simulink library "MIL_Test"  (Simulink 7.0)
values from neighbouring files (symbols this model uses):
  TID = min('TI' == AFT(1:2))    [PAS_callback.m]    (also in PSTID_callback.m = [block '/TID'])
undefined symbols (not defined in the file or in its folder): getdatatypespecs, slcm, StepSize
libraries: simulink x71, MIL_Test x6
(part 5 of 11)

== system MIL_Test/Test Data/Feature generation/Generate timed limited decrease/Subsystem/Subsystem40 ==
  In1 : Inport  OutDataType=sfix(16)  OutScaling=2^0
  In2 : Inport  Port=2  OutDataType=sfix(16)  OutScaling=2^0
  In3 : Inport  Port=3  OutDataType=sfix(16)  OutScaling=2^0
  Output1 : Sum  Inputs=|+-+  OutDataType=sfix(16)  OutScaling=2^0  SaturateOnIntegerOverflow=on  InputSameDT=on
  RO : RelationalOperator  Operator=<  LogicOutDataTypeMode=boolean
  Switch : Switch  Criteria=u2 > Threshold
  Out1 : Outport  OutDataType=sfix(16)  OutScaling=2^0
  wires:
  In3/1 -> Output1/3
  Output1/1 -> Switch/1
  RO/1 -> Switch/2
  Switch/1 -> Out1/1
  In2/1 -> RO/1, Output1/1, Switch/3  "U(k)"
  In1/1 -> RO/2, Output1/2

== system MIL_Test/Test Data/Feature generation/Generate timed limited decrease/Subsystem/Subsystem41 ==
  In1 : Inport  OutDataType=sfix(16)  OutScaling=2^0
  In2 : Inport  Port=2  OutDataType=sfix(16)  OutScaling=2^0
  In3 : Inport  Port=3  OutDataType=sfix(16)  OutScaling=2^0
  Output1 : Sum  Inputs=|+-+  OutDataType=sfix(16)  OutScaling=2^0  SaturateOnIntegerOverflow=on  InputSameDT=on
  RO : RelationalOperator  Operator=<  LogicOutDataTypeMode=boolean
  Switch : Switch  Criteria=u2 > Threshold
  Out1 : Outport  OutDataType=sfix(16)  OutScaling=2^0
  wires:
  In3/1 -> Output1/3
  Output1/1 -> Switch/1
  RO/1 -> Switch/2
  Switch/1 -> Out1/1
  In2/1 -> RO/1, Output1/1, Switch/3  "U(k)"
  In1/1 -> RO/2, Output1/2

== system MIL_Test/Test Data/Feature generation/Generate timed limited decrease/Subsystem/Subsystem42 ==
  In1 : Inport  OutDataType=sfix(16)  OutScaling=2^0
  In2 : Inport  Port=2  OutDataType=sfix(16)  OutScaling=2^0
  In3 : Inport  Port=3  OutDataType=sfix(16)  OutScaling=2^0
  Output1 : Sum  Inputs=|+-+  OutDataType=sfix(16)  OutScaling=2^0  SaturateOnIntegerOverflow=on  InputSameDT=on
  RO : RelationalOperator  Operator=<  LogicOutDataTypeMode=boolean
  Switch : Switch  Criteria=u2 > Threshold
  Out1 : Outport  OutDataType=sfix(16)  OutScaling=2^0
  wires:
  In3/1 -> Output1/3
  Output1/1 -> Switch/1
  RO/1 -> Switch/2
  Switch/1 -> Out1/1
  In2/1 -> RO/1, Output1/1, Switch/3  "U(k)"
  In1/1 -> RO/2, Output1/2

== system MIL_Test/Test Data/Feature generation/Generate timed limited decrease/Subsystem/Subsystem43 ==
  In1 : Inport  OutDataType=sfix(16)  OutScaling=2^0
  In2 : Inport  Port=2  OutDataType=sfix(16)  OutScaling=2^0
  In3 : Inport  Port=3  OutDataType=sfix(16)  OutScaling=2^0
  Output1 : Sum  Inputs=|+-+  OutDataType=sfix(16)  OutScaling=2^0  SaturateOnIntegerOverflow=on  InputSameDT=on
  RO : RelationalOperator  Operator=<  LogicOutDataTypeMode=boolean
  Switch : Switch  Criteria=u2 > Threshold
  Out1 : Outport  OutDataType=sfix(16)  OutScaling=2^0
  wires:
  In3/1 -> Output1/3
  Output1/1 -> Switch/1
  RO/1 -> Switch/2
  Switch/1 -> Out1/1
  In2/1 -> RO/1, Output1/1, Switch/3  "U(k)"
  In1/1 -> RO/2, Output1/2

== system MIL_Test/Test Data/Feature generation/Generate timed limited decrease/Subsystem/Subsystem44 ==
  In1 : Inport  OutDataType=sfix(16)  OutScaling=2^0
  In2 : Inport  Port=2  OutDataType=sfix(16)  OutScaling=2^0
  In3 : Inport  Port=3  OutDataType=sfix(16)  OutScaling=2^0
  Output1 : Sum  Inputs=|+-+  OutDataType=sfix(16)  OutScaling=2^0  SaturateOnIntegerOverflow=on  InputSameDT=on
  RO : RelationalOperator  Operator=<  LogicOutDataTypeMode=boolean
  Switch : Switch  Criteria=u2 > Threshold
  Out1 : Outport  OutDataType=sfix(16)  OutScaling=2^0
  wires:
  In3/1 -> Output1/3
  Output1/1 -> Switch/1
  RO/1 -> Switch/2
  Switch/1 -> Out1/1
  In2/1 -> RO/1, Output1/1, Switch/3  "U(k)"
  In1/1 -> RO/2, Output1/2

== system MIL_Test/Test Data/Feature generation/Generate timed limited decrease/Subsystem/Subsystem45 ==
  In1 : Inport  OutDataType=sfix(16)  OutScaling=2^0
  In2 : Inport  Port=2  OutDataType=sfix(16)  OutScaling=2^0
  In3 : Inport  Port=3  OutDataType=sfix(16)  OutScaling=2^0
  Output1 : Sum  Inputs=|+-+  OutDataType=sfix(16)  OutScaling=2^0  SaturateOnIntegerOverflow=on  InputSameDT=on
  RO : RelationalOperator  Operator=<  LogicOutDataTypeMode=boolean
  Switch : Switch  Criteria=u2 > Threshold
  Out1 : Outport  OutDataType=sfix(16)  OutScaling=2^0
  wires:
  In3/1 -> Output1/3
  Output1/1 -> Switch/1
  RO/1 -> Switch/2
  Switch/1 -> Out1/1
  In2/1 -> RO/1, Output1/1, Switch/3  "U(k)"
  In1/1 -> RO/2, Output1/2

== system MIL_Test/Test Data/Feature generation/Generate timed limited decrease/Subsystem/Subsystem46 ==
  In1 : Inport  OutDataType=sfix(16)  OutScaling=2^0
  In2 : Inport  Port=2  OutDataType=sfix(16)  OutScaling=2^0
  In3 : Inport  Port=3  OutDataType=sfix(16)  OutScaling=2^0
  Output1 : Sum  Inputs=|+-+  OutDataType=sfix(16)  OutScaling=2^0  SaturateOnIntegerOverflow=on  InputSameDT=on
  RO : RelationalOperator  Operator=<  LogicOutDataTypeMode=boolean
  Switch : Switch  Criteria=u2 > Threshold
  Out1 : Outport  OutDataType=sfix(16)  OutScaling=2^0
  wires:
  In3/1 -> Output1/3
  Output1/1 -> Switch/1
  RO/1 -> Switch/2
  Switch/1 -> Out1/1
  In2/1 -> RO/1, Output1/1, Switch/3  "U(k)"
  In1/1 -> RO/2, Output1/2

== system MIL_Test/Test Data/Feature generation/Generate timed limited decrease/Subsystem/Subsystem47 ==
  In1 : Inport  OutDataType=sfix(16)  OutScaling=2^0
  In2 : Inport  Port=2  OutDataType=sfix(16)  OutScaling=2^0
  In3 : Inport  Port=3  OutDataType=sfix(16)  OutScaling=2^0
  Output1 : Sum  Inputs=|+-+  OutDataType=sfix(16)  OutScaling=2^0  SaturateOnIntegerOverflow=on  InputSameDT=on
  RO : RelationalOperator  Operator=<  LogicOutDataTypeMode=boolean
  Switch : Switch  Criteria=u2 > Threshold
  Out1 : Outport  OutDataType=sfix(16)  OutScaling=2^0
  wires:
  In3/1 -> Output1/3
  Output1/1 -> Switch/1
  RO/1 -> Switch/2
  Switch/1 -> Out1/1
  In2/1 -> RO/1, Output1/1, Switch/3  "U(k)"
  In1/1 -> RO/2, Output1/2

== system MIL_Test/Test Data/Feature generation/Generate timed limited decrease/Subsystem/Subsystem48 ==
  In1 : Inport  OutDataType=sfix(16)  OutScaling=2^0
  In2 : Inport  Port=2  OutDataType=sfix(16)  OutScaling=2^0
  In3 : Inport  Port=3  OutDataType=sfix(16)  OutScaling=2^0
  Output1 : Sum  Inputs=|+-+  OutDataType=sfix(16)  OutScaling=2^0  SaturateOnIntegerOverflow=on  InputSameDT=on
  RO : RelationalOperator  Operator=<  LogicOutDataTypeMode=boolean
  Switch : Switch  Criteria=u2 > Threshold
  Out1 : Outport  OutDataType=sfix(16)  OutScaling=2^0
  wires:
  In3/1 -> Output1/3
  Output1/1 -> Switch/1
  RO/1 -> Switch/2
  Switch/1 -> Out1/1
  In2/1 -> RO/1, Output1/1, Switch/3  "U(k)"
  In1/1 -> RO/2, Output1/2

== system MIL_Test/Test Data/Feature generation/Generate timed limited decrease/Subsystem/Subsystem49 ==
  In1 : Inport  OutDataType=sfix(16)  OutScaling=2^0
  In2 : Inport  Port=2  OutDataType=sfix(16)  OutScaling=2^0
  In3 : Inport  Port=3  OutDataType=sfix(16)  OutScaling=2^0
  Output1 : Sum  Inputs=|+-+  OutDataType=sfix(16)  OutScaling=2^0  SaturateOnIntegerOverflow=on  InputSameDT=on
  RO : RelationalOperator  Operator=<  LogicOutDataTypeMode=boolean
  Switch : Switch  Criteria=u2 > Threshold
  Out1 : Outport  OutDataType=sfix(16)  OutScaling=2^0
  wires:
  In3/1 -> Output1/3
  Output1/1 -> Switch/1
  RO/1 -> Switch/2
  Switch/1 -> Out1/1
  In2/1 -> RO/1, Output1/1, Switch/3  "U(k)"
  In1/1 -> RO/2, Output1/2

== system MIL_Test/Test Data/Feature generation/Generate timed limited decrease/Subsystem/Subsystem5 ==
  In1 : Inport  OutDataType=sfix(16)  OutScaling=2^0
  In2 : Inport  Port=2  OutDataType=sfix(16)  OutScaling=2^0
  In3 : Inport  Port=3  OutDataType=sfix(16)  OutScaling=2^0
  Output1 : Sum  Inputs=|+-+  OutDataType=sfix(16)  OutScaling=2^0  SaturateOnIntegerOverflow=on  InputSameDT=on
  RO : RelationalOperator  Operator=<  LogicOutDataTypeMode=boolean
  Switch : Switch  Criteria=u2 > Threshold
  Out1 : Outport  OutDataType=sfix(16)  OutScaling=2^0
  wires:
  In3/1 -> Output1/3
  Output1/1 -> Switch/1
  RO/1 -> Switch/2
  Switch/1 -> Out1/1
  In2/1 -> RO/1, Output1/1, Switch/3  "U(k)"
  In1/1 -> RO/2, Output1/2

== system MIL_Test/Test Data/Feature generation/Generate timed limited decrease/Subsystem/Subsystem50 ==
  In1 : Inport  OutDataType=sfix(16)  OutScaling=2^0
  In2 : Inport  Port=2  OutDataType=sfix(16)  OutScaling=2^0
  In3 : Inport  Port=3  OutDataType=sfix(16)  OutScaling=2^0
  Output1 : Sum  Inputs=|+-+  OutDataType=sfix(16)  OutScaling=2^0  SaturateOnIntegerOverflow=on  InputSameDT=on
  RO : RelationalOperator  Operator=<  LogicOutDataTypeMode=boolean
  Switch : Switch  Criteria=u2 > Threshold
  Out1 : Outport  OutDataType=sfix(16)  OutScaling=2^0
  wires:
  In3/1 -> Output1/3
  Output1/1 -> Switch/1
  RO/1 -> Switch/2
  Switch/1 -> Out1/1
  In2/1 -> RO/1, Output1/1, Switch/3  "U(k)"
  In1/1 -> RO/2, Output1/2

== system MIL_Test/Test Data/Feature generation/Generate timed limited decrease/Subsystem/Subsystem51 ==
  In1 : Inport  OutDataType=sfix(16)  OutScaling=2^0
  In2 : Inport  Port=2  OutDataType=sfix(16)  OutScaling=2^0
  In3 : Inport  Port=3  OutDataType=sfix(16)  OutScaling=2^0
  Output1 : Sum  Inputs=|+-+  OutDataType=sfix(16)  OutScaling=2^0  SaturateOnIntegerOverflow=on  InputSameDT=on
  RO : RelationalOperator  Operator=<  LogicOutDataTypeMode=boolean
  Switch : Switch  Criteria=u2 > Threshold
  Out1 : Outport  OutDataType=sfix(16)  OutScaling=2^0
  wires:
  In3/1 -> Output1/3
  Output1/1 -> Switch/1
  RO/1 -> Switch/2
  Switch/1 -> Out1/1
  In2/1 -> RO/1, Output1/1, Switch/3  "U(k)"
  In1/1 -> RO/2, Output1/2

== system MIL_Test/Test Data/Feature generation/Generate timed limited decrease/Subsystem/Subsystem52 ==
  In1 : Inport  OutDataType=sfix(16)  OutScaling=2^0
  In2 : Inport  Port=2  OutDataType=sfix(16)  OutScaling=2^0
  In3 : Inport  Port=3  OutDataType=sfix(16)  OutScaling=2^0
  Output1 : Sum  Inputs=|+-+  OutDataType=sfix(16)  OutScaling=2^0  SaturateOnIntegerOverflow=on  InputSameDT=on
  RO : RelationalOperator  Operator=<  LogicOutDataTypeMode=boolean
  Switch : Switch  Criteria=u2 > Threshold
  Out1 : Outport  OutDataType=sfix(16)  OutScaling=2^0
  wires:
  In3/1 -> Output1/3
  Output1/1 -> Switch/1
  RO/1 -> Switch/2
  Switch/1 -> Out1/1
  In2/1 -> RO/1, Output1/1, Switch/3  "U(k)"
  In1/1 -> RO/2, Output1/2

== system MIL_Test/Test Data/Feature generation/Generate timed limited decrease/Subsystem/Subsystem53 ==
  In1 : Inport  OutDataType=sfix(16)  OutScaling=2^0
  In2 : Inport  Port=2  OutDataType=sfix(16)  OutScaling=2^0
  In3 : Inport  Port=3  OutDataType=sfix(16)  OutScaling=2^0
  Output1 : Sum  Inputs=|+-+  OutDataType=sfix(16)  OutScaling=2^0  SaturateOnIntegerOverflow=on  InputSameDT=on
  RO : RelationalOperator  Operator=<  LogicOutDataTypeMode=boolean
  Switch : Switch  Criteria=u2 > Threshold
  Out1 : Outport  OutDataType=sfix(16)  OutScaling=2^0
  wires:
  In3/1 -> Output1/3
  Output1/1 -> Switch/1
  RO/1 -> Switch/2
  Switch/1 -> Out1/1
  In2/1 -> RO/1, Output1/1, Switch/3  "U(k)"
  In1/1 -> RO/2, Output1/2

== system MIL_Test/Test Data/Feature generation/Generate timed limited decrease/Subsystem/Subsystem54 ==
  In1 : Inport  OutDataType=sfix(16)  OutScaling=2^0
  In2 : Inport  Port=2  OutDataType=sfix(16)  OutScaling=2^0
  In3 : Inport  Port=3  OutDataType=sfix(16)  OutScaling=2^0
  Output1 : Sum  Inputs=|+-+  OutDataType=sfix(16)  OutScaling=2^0  SaturateOnIntegerOverflow=on  InputSameDT=on
  RO : RelationalOperator  Operator=<  LogicOutDataTypeMode=boolean
  Switch : Switch  Criteria=u2 > Threshold
  Out1 : Outport  OutDataType=sfix(16)  OutScaling=2^0
  wires:
  In3/1 -> Output1/3
  Output1/1 -> Switch/1
  RO/1 -> Switch/2
  Switch/1 -> Out1/1
  In2/1 -> RO/1, Output1/1, Switch/3  "U(k)"
  In1/1 -> RO/2, Output1/2

== system MIL_Test/Test Data/Feature generation/Generate timed limited decrease/Subsystem/Subsystem55 ==
  In1 : Inport  OutDataType=sfix(16)  OutScaling=2^0
  In2 : Inport  Port=2  OutDataType=sfix(16)  OutScaling=2^0
  In3 : Inport  Port=3  OutDataType=sfix(16)  OutScaling=2^0
  Output1 : Sum  Inputs=|+-+  OutDataType=sfix(16)  OutScaling=2^0  SaturateOnIntegerOverflow=on  InputSameDT=on
  RO : RelationalOperator  Operator=<  LogicOutDataTypeMode=boolean
  Switch : Switch  Criteria=u2 > Threshold
  Out1 : Outport  OutDataType=sfix(16)  OutScaling=2^0
  wires:
  In3/1 -> Output1/3
  Output1/1 -> Switch/1
  RO/1 -> Switch/2
  Switch/1 -> Out1/1
  In2/1 -> RO/1, Output1/1, Switch/3  "U(k)"
  In1/1 -> RO/2, Output1/2

== system MIL_Test/Test Data/Feature generation/Generate timed limited decrease/Subsystem/Subsystem56 ==
  In1 : Inport  OutDataType=sfix(16)  OutScaling=2^0
  In2 : Inport  Port=2  OutDataType=sfix(16)  OutScaling=2^0
  In3 : Inport  Port=3  OutDataType=sfix(16)  OutScaling=2^0
  Output1 : Sum  Inputs=|+-+  OutDataType=sfix(16)  OutScaling=2^0  SaturateOnIntegerOverflow=on  InputSameDT=on
  RO : RelationalOperator  Operator=<  LogicOutDataTypeMode=boolean
  Switch : Switch  Criteria=u2 > Threshold
  Out1 : Outport  OutDataType=sfix(16)  OutScaling=2^0
  wires:
  In3/1 -> Output1/3
  Output1/1 -> Switch/1
  RO/1 -> Switch/2
  Switch/1 -> Out1/1
  In2/1 -> RO/1, Output1/1, Switch/3  "U(k)"
  In1/1 -> RO/2, Output1/2

== system MIL_Test/Test Data/Feature generation/Generate timed limited decrease/Subsystem/Subsystem57 ==
  In1 : Inport  OutDataType=sfix(16)  OutScaling=2^0
  In2 : Inport  Port=2  OutDataType=sfix(16)  OutScaling=2^0
  In3 : Inport  Port=3  OutDataType=sfix(16)  OutScaling=2^0
  Output1 : Sum  Inputs=|+-+  OutDataType=sfix(16)  OutScaling=2^0  SaturateOnIntegerOverflow=on  InputSameDT=on
  RO : RelationalOperator  Operator=<  LogicOutDataTypeMode=boolean
  Switch : Switch  Criteria=u2 > Threshold
  Out1 : Outport  OutDataType=sfix(16)  OutScaling=2^0
  wires:
  In3/1 -> Output1/3
  Output1/1 -> Switch/1
  RO/1 -> Switch/2
  Switch/1 -> Out1/1
  In2/1 -> RO/1, Output1/1, Switch/3  "U(k)"
  In1/1 -> RO/2, Output1/2

== system MIL_Test/Test Data/Feature generation/Generate timed limited decrease/Subsystem/Subsystem58 ==
  In1 : Inport  OutDataType=sfix(16)  OutScaling=2^0
  In2 : Inport  Port=2  OutDataType=sfix(16)  OutScaling=2^0
  In3 : Inport  Port=3  OutDataType=sfix(16)  OutScaling=2^0
  Output1 : Sum  Inputs=|+-+  OutDataType=sfix(16)  OutScaling=2^0  SaturateOnIntegerOverflow=on  InputSameDT=on
  RO : RelationalOperator  Operator=<  LogicOutDataTypeMode=boolean
  Switch : Switch  Criteria=u2 > Threshold
  Out1 : Outport  OutDataType=sfix(16)  OutScaling=2^0
  wires:
  In3/1 -> Output1/3
  Output1/1 -> Switch/1
  RO/1 -> Switch/2
  Switch/1 -> Out1/1
  In2/1 -> RO/1, Output1/1, Switch/3  "U(k)"
  In1/1 -> RO/2, Output1/2

== system MIL_Test/Test Data/Feature generation/Generate timed limited decrease/Subsystem/Subsystem59 ==
  In1 : Inport  OutDataType=sfix(16)  OutScaling=2^0
  In2 : Inport  Port=2  OutDataType=sfix(16)  OutScaling=2^0
  In3 : Inport  Port=3  OutDataType=sfix(16)  OutScaling=2^0
  Output1 : Sum  Inputs=|+-+  OutDataType=sfix(16)  OutScaling=2^0  SaturateOnIntegerOverflow=on  InputSameDT=on
  RO : RelationalOperator  Operator=<  LogicOutDataTypeMode=boolean
  Switch : Switch  Criteria=u2 > Threshold
  Out1 : Outport  OutDataType=sfix(16)  OutScaling=2^0
  wires:
  In3/1 -> Output1/3
  Output1/1 -> Switch/1
  RO/1 -> Switch/2
  Switch/1 -> Out1/1
  In2/1 -> RO/1, Output1/1, Switch/3  "U(k)"
  In1/1 -> RO/2, Output1/2

== system MIL_Test/Test Data/Feature generation/Generate timed limited decrease/Subsystem/Subsystem6 ==
  In1 : Inport  OutDataType=sfix(16)  OutScaling=2^0
  In2 : Inport  Port=2  OutDataType=sfix(16)  OutScaling=2^0
  In3 : Inport  Port=3  OutDataType=sfix(16)  OutScaling=2^0
  Output1 : Sum  Inputs=|+-+  OutDataType=sfix(16)  OutScaling=2^0  SaturateOnIntegerOverflow=on  InputSameDT=on
  RO : RelationalOperator  Operator=<  LogicOutDataTypeMode=boolean
  Switch : Switch  Criteria=u2 > Threshold
  Out1 : Outport  OutDataType=sfix(16)  OutScaling=2^0
  wires:
  In3/1 -> Output1/3
  Output1/1 -> Switch/1
  RO/1 -> Switch/2
  Switch/1 -> Out1/1
  In2/1 -> RO/1, Output1/1, Switch/3  "U(k)"
  In1/1 -> RO/2, Output1/2

== system MIL_Test/Test Data/Feature generation/Generate timed limited decrease/Subsystem/Subsystem60 ==
  In1 : Inport  OutDataType=sfix(16)  OutScaling=2^0
  In2 : Inport  Port=2  OutDataType=sfix(16)  OutScaling=2^0
  In3 : Inport  Port=3  OutDataType=sfix(16)  OutScaling=2^0
  Output1 : Sum  Inputs=|+-+  OutDataType=sfix(16)  OutScaling=2^0  SaturateOnIntegerOverflow=on  InputSameDT=on
  RO : RelationalOperator  Operator=<  LogicOutDataTypeMode=boolean
  Switch : Switch  Criteria=u2 > Threshold
  Out1 : Outport  OutDataType=sfix(16)  OutScaling=2^0
  wires:
  In3/1 -> Output1/3
  Output1/1 -> Switch/1
  RO/1 -> Switch/2
  Switch/1 -> Out1/1
  In2/1 -> RO/1, Output1/1, Switch/3  "U(k)"
  In1/1 -> RO/2, Output1/2

== system MIL_Test/Test Data/Feature generation/Generate timed limited decrease/Subsystem/Subsystem61 ==
  In1 : Inport  OutDataType=sfix(16)  OutScaling=2^0
  In2 : Inport  Port=2  OutDataType=sfix(16)  OutScaling=2^0
  In3 : Inport  Port=3  OutDataType=sfix(16)  OutScaling=2^0
  Output1 : Sum  Inputs=|+-+  OutDataType=sfix(16)  OutScaling=2^0  SaturateOnIntegerOverflow=on  InputSameDT=on
  RO : RelationalOperator  Operator=<  LogicOutDataTypeMode=boolean
  Switch : Switch  Criteria=u2 > Threshold
  Out1 : Outport  OutDataType=sfix(16)  OutScaling=2^0
  wires:
  In3/1 -> Output1/3
  Output1/1 -> Switch/1
  RO/1 -> Switch/2
  Switch/1 -> Out1/1
  In2/1 -> RO/1, Output1/1, Switch/3  "U(k)"
  In1/1 -> RO/2, Output1/2

== system MIL_Test/Test Data/Feature generation/Generate timed limited decrease/Subsystem/Subsystem62 ==
  In1 : Inport  OutDataType=sfix(16)  OutScaling=2^0
  In2 : Inport  Port=2  OutDataType=sfix(16)  OutScaling=2^0
  In3 : Inport  Port=3  OutDataType=sfix(16)  OutScaling=2^0
  Output1 : Sum  Inputs=|+-+  OutDataType=sfix(16)  OutScaling=2^0  SaturateOnIntegerOverflow=on  InputSameDT=on
  RO : RelationalOperator  Operator=<  LogicOutDataTypeMode=boolean
  Switch : Switch  Criteria=u2 > Threshold
  Out1 : Outport  OutDataType=sfix(16)  OutScaling=2^0
  wires:
  In3/1 -> Output1/3
  Output1/1 -> Switch/1
  RO/1 -> Switch/2
  Switch/1 -> Out1/1
  In2/1 -> RO/1, Output1/1, Switch/3  "U(k)"
  In1/1 -> RO/2, Output1/2

== system MIL_Test/Test Data/Feature generation/Generate timed limited decrease/Subsystem/Subsystem63 ==
  In1 : Inport  OutDataType=sfix(16)  OutScaling=2^0
  In2 : Inport  Port=2  OutDataType=sfix(16)  OutScaling=2^0
  In3 : Inport  Port=3  OutDataType=sfix(16)  OutScaling=2^0
  Output1 : Sum  Inputs=|+-+  OutDataType=sfix(16)  OutScaling=2^0  SaturateOnIntegerOverflow=on  InputSameDT=on
  RO : RelationalOperator  Operator=<  LogicOutDataTypeMode=boolean
  Switch : Switch  Criteria=u2 > Threshold
  Out1 : Outport  OutDataType=sfix(16)  OutScaling=2^0
  wires:
  In3/1 -> Output1/3
  Output1/1 -> Switch/1
  RO/1 -> Switch/2
  Switch/1 -> Out1/1
  In2/1 -> RO/1, Output1/1, Switch/3  "U(k)"
  In1/1 -> RO/2, Output1/2

== system MIL_Test/Test Data/Feature generation/Generate timed limited decrease/Subsystem/Subsystem64 ==
  In1 : Inport  OutDataType=sfix(16)  OutScaling=2^0
  In2 : Inport  Port=2  OutDataType=sfix(16)  OutScaling=2^0
  In3 : Inport  Port=3  OutDataType=sfix(16)  OutScaling=2^0
  Output1 : Sum  Inputs=|+-+  OutDataType=sfix(16)  OutScaling=2^0  SaturateOnIntegerOverflow=on  InputSameDT=on
  RO : RelationalOperator  Operator=<  LogicOutDataTypeMode=boolean
  Switch : Switch  Criteria=u2 > Threshold
  Out1 : Outport  OutDataType=sfix(16)  OutScaling=2^0
  wires:
  In3/1 -> Output1/3
  Output1/1 -> Switch/1
  RO/1 -> Switch/2
  Switch/1 -> Out1/1
  In2/1 -> RO/1, Output1/1, Switch/3  "U(k)"
  In1/1 -> RO/2, Output1/2

== system MIL_Test/Test Data/Feature generation/Generate timed limited decrease/Subsystem/Subsystem65 ==
  In1 : Inport  OutDataType=sfix(16)  OutScaling=2^0
  In2 : Inport  Port=2  OutDataType=sfix(16)  OutScaling=2^0
  In3 : Inport  Port=3  OutDataType=sfix(16)  OutScaling=2^0
  Output1 : Sum  Inputs=|+-+  OutDataType=sfix(16)  OutScaling=2^0  SaturateOnIntegerOverflow=on  InputSameDT=on
  RO : RelationalOperator  Operator=<  LogicOutDataTypeMode=boolean
  Switch : Switch  Criteria=u2 > Threshold
  Out1 : Outport  OutDataType=sfix(16)  OutScaling=2^0
  wires:
  In3/1 -> Output1/3
  Output1/1 -> Switch/1
  RO/1 -> Switch/2
  Switch/1 -> Out1/1
  In2/1 -> RO/1, Output1/1, Switch/3  "U(k)"
  In1/1 -> RO/2, Output1/2

== system MIL_Test/Test Data/Feature generation/Generate timed limited decrease/Subsystem/Subsystem66 ==
  In1 : Inport  OutDataType=sfix(16)  OutScaling=2^0
  In2 : Inport  Port=2  OutDataType=sfix(16)  OutScaling=2^0
  In3 : Inport  Port=3  OutDataType=sfix(16)  OutScaling=2^0
  Output1 : Sum  Inputs=|+-+  OutDataType=sfix(16)  OutScaling=2^0  SaturateOnIntegerOverflow=on  InputSameDT=on
  RO : RelationalOperator  Operator=<  LogicOutDataTypeMode=boolean
  Switch : Switch  Criteria=u2 > Threshold
  Out1 : Outport  OutDataType=sfix(16)  OutScaling=2^0
  wires:
  In3/1 -> Output1/3
  Output1/1 -> Switch/1
  RO/1 -> Switch/2
  Switch/1 -> Out1/1
  In2/1 -> RO/1, Output1/1, Switch/3  "U(k)"
  In1/1 -> RO/2, Output1/2

== system MIL_Test/Test Data/Feature generation/Generate timed limited decrease/Subsystem/Subsystem67 ==
  In1 : Inport  OutDataType=sfix(16)  OutScaling=2^0
  In2 : Inport  Port=2  OutDataType=sfix(16)  OutScaling=2^0
  In3 : Inport  Port=3  OutDataType=sfix(16)  OutScaling=2^0
  Output1 : Sum  Inputs=|+-+  OutDataType=sfix(16)  OutScaling=2^0  SaturateOnIntegerOverflow=on  InputSameDT=on
  RO : RelationalOperator  Operator=<  LogicOutDataTypeMode=boolean
  Switch : Switch  Criteria=u2 > Threshold
  Out1 : Outport  OutDataType=sfix(16)  OutScaling=2^0
  wires:
  In3/1 -> Output1/3
  Output1/1 -> Switch/1
  RO/1 -> Switch/2
  Switch/1 -> Out1/1
  In2/1 -> RO/1, Output1/1, Switch/3  "U(k)"
  In1/1 -> RO/2, Output1/2

== system MIL_Test/Test Data/Feature generation/Generate timed limited decrease/Subsystem/Subsystem68 ==
  In1 : Inport  OutDataType=sfix(16)  OutScaling=2^0
  In2 : Inport  Port=2  OutDataType=sfix(16)  OutScaling=2^0
  In3 : Inport  Port=3  OutDataType=sfix(16)  OutScaling=2^0
  Output1 : Sum  Inputs=|+-+  OutDataType=sfix(16)  OutScaling=2^0  SaturateOnIntegerOverflow=on  InputSameDT=on
  RO : RelationalOperator  Operator=<  LogicOutDataTypeMode=boolean
  Switch : Switch  Criteria=u2 > Threshold
  Out1 : Outport  OutDataType=sfix(16)  OutScaling=2^0
  wires:
  In3/1 -> Output1/3
  Output1/1 -> Switch/1
  RO/1 -> Switch/2
  Switch/1 -> Out1/1
  In2/1 -> RO/1, Output1/1, Switch/3  "U(k)"
  In1/1 -> RO/2, Output1/2

== system MIL_Test/Test Data/Feature generation/Generate timed limited decrease/Subsystem/Subsystem69 ==
  In1 : Inport  OutDataType=sfix(16)  OutScaling=2^0
  In2 : Inport  Port=2  OutDataType=sfix(16)  OutScaling=2^0
  In3 : Inport  Port=3  OutDataType=sfix(16)  OutScaling=2^0
  Output1 : Sum  Inputs=|+-+  OutDataType=sfix(16)  OutScaling=2^0  SaturateOnIntegerOverflow=on  InputSameDT=on
  RO : RelationalOperator  Operator=<  LogicOutDataTypeMode=boolean
  Switch : Switch  Criteria=u2 > Threshold
  Out1 : Outport  OutDataType=sfix(16)  OutScaling=2^0
  wires:
  In3/1 -> Output1/3
  Output1/1 -> Switch/1
  RO/1 -> Switch/2
  Switch/1 -> Out1/1
  In2/1 -> RO/1, Output1/1, Switch/3  "U(k)"
  In1/1 -> RO/2, Output1/2

== system MIL_Test/Test Data/Feature generation/Generate timed limited decrease/Subsystem/Subsystem7 ==
  In1 : Inport  OutDataType=sfix(16)  OutScaling=2^0
  In2 : Inport  Port=2  OutDataType=sfix(16)  OutScaling=2^0
  In3 : Inport  Port=3  OutDataType=sfix(16)  OutScaling=2^0
  Output1 : Sum  Inputs=|+-+  OutDataType=sfix(16)  OutScaling=2^0  SaturateOnIntegerOverflow=on  InputSameDT=on
  RO : RelationalOperator  Operator=<  LogicOutDataTypeMode=boolean
  Switch : Switch  Criteria=u2 > Threshold
  Out1 : Outport  OutDataType=sfix(16)  OutScaling=2^0
  wires:
  In3/1 -> Output1/3
  Output1/1 -> Switch/1
  RO/1 -> Switch/2
  Switch/1 -> Out1/1
  In2/1 -> RO/1, Output1/1, Switch/3  "U(k)"
  In1/1 -> RO/2, Output1/2

== system MIL_Test/Test Data/Feature generation/Generate timed limited decrease/Subsystem/Subsystem70 ==
  In1 : Inport  OutDataType=sfix(16)  OutScaling=2^0
  In2 : Inport  Port=2  OutDataType=sfix(16)  OutScaling=2^0
  In3 : Inport  Port=3  OutDataType=sfix(16)  OutScaling=2^0
  Output1 : Sum  Inputs=|+-+  OutDataType=sfix(16)  OutScaling=2^0  SaturateOnIntegerOverflow=on  InputSameDT=on
  RO : RelationalOperator  Operator=<  LogicOutDataTypeMode=boolean
  Switch : Switch  Criteria=u2 > Threshold
  Out1 : Outport  OutDataType=sfix(16)  OutScaling=2^0
  wires:
  In3/1 -> Output1/3
  Output1/1 -> Switch/1
  RO/1 -> Switch/2
  Switch/1 -> Out1/1
  In2/1 -> RO/1, Output1/1, Switch/3  "U(k)"
  In1/1 -> RO/2, Output1/2

== system MIL_Test/Test Data/Feature generation/Generate timed limited decrease/Subsystem/Subsystem8 ==
  In1 : Inport  OutDataType=sfix(16)  OutScaling=2^0
  In2 : Inport  Port=2  OutDataType=sfix(16)  OutScaling=2^0
  In3 : Inport  Port=3  OutDataType=sfix(16)  OutScaling=2^0
  Output1 : Sum  Inputs=|+-+  OutDataType=sfix(16)  OutScaling=2^0  SaturateOnIntegerOverflow=on  InputSameDT=on
  RO : RelationalOperator  Operator=<  LogicOutDataTypeMode=boolean
  Switch : Switch  Criteria=u2 > Threshold
  Out1 : Outport  OutDataType=sfix(16)  OutScaling=2^0
  wires:
  In3/1 -> Output1/3
  Output1/1 -> Switch/1
  RO/1 -> Switch/2
  Switch/1 -> Out1/1
  In2/1 -> RO/1, Output1/1, Switch/3  "U(k)"
  In1/1 -> RO/2, Output1/2

== system MIL_Test/Test Data/Feature generation/Generate timed limited decrease/Subsystem/Subsystem9 ==
  In1 : Inport  OutDataType=sfix(16)  OutScaling=2^0
  In2 : Inport  Port=2  OutDataType=sfix(16)  OutScaling=2^0
  In3 : Inport  Port=3  OutDataType=sfix(16)  OutScaling=2^0
  Output1 : Sum  Inputs=|+-+  OutDataType=sfix(16)  OutScaling=2^0  SaturateOnIntegerOverflow=on  InputSameDT=on
  RO : RelationalOperator  Operator=<  LogicOutDataTypeMode=boolean
  Switch : Switch  Criteria=u2 > Threshold
  Out1 : Outport  OutDataType=sfix(16)  OutScaling=2^0
  wires:
  In3/1 -> Output1/3
  Output1/1 -> Switch/1
  RO/1 -> Switch/2
  Switch/1 -> Out1/1
  In2/1 -> RO/1, Output1/1, Switch/3  "U(k)"
  In1/1 -> RO/2, Output1/2

== system MIL_Test/Test Data/Feature generation/Generate timed limited increase/Subsystem/Subsystem1 ==
  In1 : Inport  OutDataType=sfix(16)  OutScaling=2^0
  In2 : Inport  Port=2  OutDataType=sfix(16)  OutScaling=2^0
  In3 : Inport  Port=3  OutDataType=sfix(16)  OutScaling=2^0
  Output1 : Sum  Inputs=|+-+  OutDataType=sfix(16)  OutScaling=2^0  SaturateOnIntegerOverflow=on  InputSameDT=on
  RO : RelationalOperator  Operator=>  LogicOutDataTypeMode=boolean
  Switch : Switch  Criteria=u2 > Threshold
  Out1 : Outport  OutDataType=sfix(16)  OutScaling=2^0
  wires:
  In3/1 -> Output1/3
  Output1/1 -> Switch/1
  RO/1 -> Switch/2
  Switch/1 -> Out1/1
  In2/1 -> RO/1, Output1/1, Switch/3  "U(k)"
  In1/1 -> RO/2, Output1/2

== system MIL_Test/Test Data/Feature generation/Generate timed limited increase/Subsystem/Subsystem10 ==
  In1 : Inport  OutDataType=sfix(16)  OutScaling=2^0
  In2 : Inport  Port=2  OutDataType=sfix(16)  OutScaling=2^0
  In3 : Inport  Port=3  OutDataType=sfix(16)  OutScaling=2^0
  Output1 : Sum  Inputs=|+-+  OutDataType=sfix(16)  OutScaling=2^0  SaturateOnIntegerOverflow=on  InputSameDT=on
  RO : RelationalOperator  Operator=>  LogicOutDataTypeMode=boolean
  Switch : Switch  Criteria=u2 > Threshold
  Out1 : Outport  OutDataType=sfix(16)  OutScaling=2^0
  wires:
  In3/1 -> Output1/3
  Output1/1 -> Switch/1
  RO/1 -> Switch/2
  Switch/1 -> Out1/1
  In2/1 -> RO/1, Output1/1, Switch/3  "U(k)"
  In1/1 -> RO/2, Output1/2

== system MIL_Test/Test Data/Feature generation/Generate timed limited increase/Subsystem/Subsystem11 ==
  In1 : Inport  OutDataType=sfix(16)  OutScaling=2^0
  In2 : Inport  Port=2  OutDataType=sfix(16)  OutScaling=2^0
  In3 : Inport  Port=3  OutDataType=sfix(16)  OutScaling=2^0
  Output1 : Sum  Inputs=|+-+  OutDataType=sfix(16)  OutScaling=2^0  SaturateOnIntegerOverflow=on  InputSameDT=on
  RO : RelationalOperator  Operator=>  LogicOutDataTypeMode=boolean
  Switch : Switch  Criteria=u2 > Threshold
  Out1 : Outport  OutDataType=sfix(16)  OutScaling=2^0
  wires:
  In3/1 -> Output1/3
  Output1/1 -> Switch/1
  RO/1 -> Switch/2
  Switch/1 -> Out1/1
  In2/1 -> RO/1, Output1/1, Switch/3  "U(k)"
  In1/1 -> RO/2, Output1/2

== system MIL_Test/Test Data/Feature generation/Generate timed limited increase/Subsystem/Subsystem12 ==
  In1 : Inport  OutDataType=sfix(16)  OutScaling=2^0
  In2 : Inport  Port=2  OutDataType=sfix(16)  OutScaling=2^0
  In3 : Inport  Port=3  OutDataType=sfix(16)  OutScaling=2^0
  Output1 : Sum  Inputs=|+-+  OutDataType=sfix(16)  OutScaling=2^0  SaturateOnIntegerOverflow=on  InputSameDT=on
  RO : RelationalOperator  Operator=>  LogicOutDataTypeMode=boolean
  Switch : Switch  Criteria=u2 > Threshold
  Out1 : Outport  OutDataType=sfix(16)  OutScaling=2^0
  wires:
  In3/1 -> Output1/3
  Output1/1 -> Switch/1
  RO/1 -> Switch/2
  Switch/1 -> Out1/1
  In2/1 -> RO/1, Output1/1, Switch/3  "U(k)"
  In1/1 -> RO/2, Output1/2

== system MIL_Test/Test Data/Feature generation/Generate timed limited increase/Subsystem/Subsystem13 ==
  In1 : Inport  OutDataType=sfix(16)  OutScaling=2^0
  In2 : Inport  Port=2  OutDataType=sfix(16)  OutScaling=2^0
  In3 : Inport  Port=3  OutDataType=sfix(16)  OutScaling=2^0
  Output1 : Sum  Inputs=|+-+  OutDataType=sfix(16)  OutScaling=2^0  SaturateOnIntegerOverflow=on  InputSameDT=on
  RO : RelationalOperator  Operator=>  LogicOutDataTypeMode=boolean
  Switch : Switch  Criteria=u2 > Threshold
  Out1 : Outport  OutDataType=sfix(16)  OutScaling=2^0
  wires:
  In3/1 -> Output1/3
  Output1/1 -> Switch/1
  RO/1 -> Switch/2
  Switch/1 -> Out1/1
  In2/1 -> RO/1, Output1/1, Switch/3  "U(k)"
  In1/1 -> RO/2, Output1/2

== system MIL_Test/Test Data/Feature generation/Generate timed limited increase/Subsystem/Subsystem14 ==
  In1 : Inport  OutDataType=sfix(16)  OutScaling=2^0
  In2 : Inport  Port=2  OutDataType=sfix(16)  OutScaling=2^0
  In3 : Inport  Port=3  OutDataType=sfix(16)  OutScaling=2^0
  Output1 : Sum  Inputs=|+-+  OutDataType=sfix(16)  OutScaling=2^0  SaturateOnIntegerOverflow=on  InputSameDT=on
  RO : RelationalOperator  Operator=>  LogicOutDataTypeMode=boolean
  Switch : Switch  Criteria=u2 > Threshold
  Out1 : Outport  OutDataType=sfix(16)  OutScaling=2^0
  wires:
  In3/1 -> Output1/3
  Output1/1 -> Switch/1
  RO/1 -> Switch/2
  Switch/1 -> Out1/1
  In2/1 -> RO/1, Output1/1, Switch/3  "U(k)"
  In1/1 -> RO/2, Output1/2

== system MIL_Test/Test Data/Feature generation/Generate timed limited increase/Subsystem/Subsystem15 ==
  In1 : Inport  OutDataType=sfix(16)  OutScaling=2^0
  In2 : Inport  Port=2  OutDataType=sfix(16)  OutScaling=2^0
  In3 : Inport  Port=3  OutDataType=sfix(16)  OutScaling=2^0
  Output1 : Sum  Inputs=|+-+  OutDataType=sfix(16)  OutScaling=2^0  SaturateOnIntegerOverflow=on  InputSameDT=on
  RO : RelationalOperator  Operator=>  LogicOutDataTypeMode=boolean
  Switch : Switch  Criteria=u2 > Threshold
  Out1 : Outport  OutDataType=sfix(16)  OutScaling=2^0
  wires:
  In3/1 -> Output1/3
  Output1/1 -> Switch/1
  RO/1 -> Switch/2
  Switch/1 -> Out1/1
  In2/1 -> RO/1, Output1/1, Switch/3  "U(k)"
  In1/1 -> RO/2, Output1/2

== system MIL_Test/Test Data/Feature generation/Generate timed limited increase/Subsystem/Subsystem16 ==
  In1 : Inport  OutDataType=sfix(16)  OutScaling=2^0
  In2 : Inport  Port=2  OutDataType=sfix(16)  OutScaling=2^0
  In3 : Inport  Port=3  OutDataType=sfix(16)  OutScaling=2^0
  Output1 : Sum  Inputs=|+-+  OutDataType=sfix(16)  OutScaling=2^0  SaturateOnIntegerOverflow=on  InputSameDT=on
  RO : RelationalOperator  Operator=>  LogicOutDataTypeMode=boolean
  Switch : Switch  Criteria=u2 > Threshold
  Out1 : Outport  OutDataType=sfix(16)  OutScaling=2^0
  wires:
  In3/1 -> Output1/3
  Output1/1 -> Switch/1
  RO/1 -> Switch/2
  Switch/1 -> Out1/1
  In2/1 -> RO/1, Output1/1, Switch/3  "U(k)"
  In1/1 -> RO/2, Output1/2

== system MIL_Test/Test Data/Feature generation/Generate timed limited increase/Subsystem/Subsystem17 ==
  In1 : Inport  OutDataType=sfix(16)  OutScaling=2^0
  In2 : Inport  Port=2  OutDataType=sfix(16)  OutScaling=2^0
  In3 : Inport  Port=3  OutDataType=sfix(16)  OutScaling=2^0
  Output1 : Sum  Inputs=|+-+  OutDataType=sfix(16)  OutScaling=2^0  SaturateOnIntegerOverflow=on  InputSameDT=on
  RO : RelationalOperator  Operator=>  LogicOutDataTypeMode=boolean
  Switch : Switch  Criteria=u2 > Threshold
  Out1 : Outport  OutDataType=sfix(16)  OutScaling=2^0
  wires:
  In3/1 -> Output1/3
  Output1/1 -> Switch/1
  RO/1 -> Switch/2
  Switch/1 -> Out1/1
  In2/1 -> RO/1, Output1/1, Switch/3  "U(k)"
  In1/1 -> RO/2, Output1/2

== system MIL_Test/Test Data/Feature generation/Generate timed limited increase/Subsystem/Subsystem18 ==
  In1 : Inport  OutDataType=sfix(16)  OutScaling=2^0
  In2 : Inport  Port=2  OutDataType=sfix(16)  OutScaling=2^0
  In3 : Inport  Port=3  OutDataType=sfix(16)  OutScaling=2^0
  Output1 : Sum  Inputs=|+-+  OutDataType=sfix(16)  OutScaling=2^0  SaturateOnIntegerOverflow=on  InputSameDT=on
  RO : RelationalOperator  Operator=>  LogicOutDataTypeMode=boolean
  Switch : Switch  Criteria=u2 > Threshold
  Out1 : Outport  OutDataType=sfix(16)  OutScaling=2^0
  wires:
  In3/1 -> Output1/3
  Output1/1 -> Switch/1
  RO/1 -> Switch/2
  Switch/1 -> Out1/1
  In2/1 -> RO/1, Output1/1, Switch/3  "U(k)"
  In1/1 -> RO/2, Output1/2

== system MIL_Test/Test Data/Feature generation/Generate timed limited increase/Subsystem/Subsystem19 ==
  In1 : Inport  OutDataType=sfix(16)  OutScaling=2^0
  In2 : Inport  Port=2  OutDataType=sfix(16)  OutScaling=2^0
  In3 : Inport  Port=3  OutDataType=sfix(16)  OutScaling=2^0
  Output1 : Sum  Inputs=|+-+  OutDataType=sfix(16)  OutScaling=2^0  SaturateOnIntegerOverflow=on  InputSameDT=on
  RO : RelationalOperator  Operator=>  LogicOutDataTypeMode=boolean
  Switch : Switch  Criteria=u2 > Threshold
  Out1 : Outport  OutDataType=sfix(16)  OutScaling=2^0
  wires:
  In3/1 -> Output1/3
  Output1/1 -> Switch/1
  RO/1 -> Switch/2
  Switch/1 -> Out1/1
  In2/1 -> RO/1, Output1/1, Switch/3  "U(k)"
  In1/1 -> RO/2, Output1/2

== system MIL_Test/Test Data/Feature generation/Generate timed limited increase/Subsystem/Subsystem2 ==
  In1 : Inport  OutDataType=sfix(16)  OutScaling=2^0
  In2 : Inport  Port=2  OutDataType=sfix(16)  OutScaling=2^0
  In3 : Inport  Port=3  OutDataType=sfix(16)  OutScaling=2^0
  Output1 : Sum  Inputs=|+-+  OutDataType=sfix(16)  OutScaling=2^0  SaturateOnIntegerOverflow=on  InputSameDT=on
  RO : RelationalOperator  Operator=>  LogicOutDataTypeMode=boolean
  Switch : Switch  Criteria=u2 > Threshold
  Out1 : Outport  OutDataType=sfix(16)  OutScaling=2^0
  wires:
  In3/1 -> Output1/3
  Output1/1 -> Switch/1
  RO/1 -> Switch/2
  Switch/1 -> Out1/1
  In2/1 -> RO/1, Output1/1, Switch/3  "U(k)"
  In1/1 -> RO/2, Output1/2

== system MIL_Test/Test Data/Feature generation/Generate timed limited increase/Subsystem/Subsystem20 ==
  In1 : Inport  OutDataType=sfix(16)  OutScaling=2^0
  In2 : Inport  Port=2  OutDataType=sfix(16)  OutScaling=2^0
  In3 : Inport  Port=3  OutDataType=sfix(16)  OutScaling=2^0
  Output1 : Sum  Inputs=|+-+  OutDataType=sfix(16)  OutScaling=2^0  SaturateOnIntegerOverflow=on  InputSameDT=on
  RO : RelationalOperator  Operator=>  LogicOutDataTypeMode=boolean
  Switch : Switch  Criteria=u2 > Threshold
  Out1 : Outport  OutDataType=sfix(16)  OutScaling=2^0
  wires:
  In3/1 -> Output1/3
  Output1/1 -> Switch/1
  RO/1 -> Switch/2
  Switch/1 -> Out1/1
  In2/1 -> RO/1, Output1/1, Switch/3  "U(k)"
  In1/1 -> RO/2, Output1/2

== system MIL_Test/Test Data/Feature generation/Generate timed limited increase/Subsystem/Subsystem21 ==
  In1 : Inport  OutDataType=sfix(16)  OutScaling=2^0
  In2 : Inport  Port=2  OutDataType=sfix(16)  OutScaling=2^0
  In3 : Inport  Port=3  OutDataType=sfix(16)  OutScaling=2^0
  Output1 : Sum  Inputs=|+-+  OutDataType=sfix(16)  OutScaling=2^0  SaturateOnIntegerOverflow=on  InputSameDT=on
  RO : RelationalOperator  Operator=>  LogicOutDataTypeMode=boolean
  Switch : Switch  Criteria=u2 > Threshold
  Out1 : Outport  OutDataType=sfix(16)  OutScaling=2^0
  wires:
  In3/1 -> Output1/3
  Output1/1 -> Switch/1
  RO/1 -> Switch/2
  Switch/1 -> Out1/1
  In2/1 -> RO/1, Output1/1, Switch/3  "U(k)"
  In1/1 -> RO/2, Output1/2

== system MIL_Test/Test Data/Feature generation/Generate timed limited increase/Subsystem/Subsystem22 ==
  In1 : Inport  OutDataType=sfix(16)  OutScaling=2^0
  In2 : Inport  Port=2  OutDataType=sfix(16)  OutScaling=2^0
  In3 : Inport  Port=3  OutDataType=sfix(16)  OutScaling=2^0
  Output1 : Sum  Inputs=|+-+  OutDataType=sfix(16)  OutScaling=2^0  SaturateOnIntegerOverflow=on  InputSameDT=on
  RO : RelationalOperator  Operator=>  LogicOutDataTypeMode=boolean
  Switch : Switch  Criteria=u2 > Threshold
  Out1 : Outport  OutDataType=sfix(16)  OutScaling=2^0
  wires:
  In3/1 -> Output1/3
  Output1/1 -> Switch/1
  RO/1 -> Switch/2
  Switch/1 -> Out1/1
  In2/1 -> RO/1, Output1/1, Switch/3  "U(k)"
  In1/1 -> RO/2, Output1/2

== system MIL_Test/Test Data/Feature generation/Generate timed limited increase/Subsystem/Subsystem23 ==
  In1 : Inport  OutDataType=sfix(16)  OutScaling=2^0
  In2 : Inport  Port=2  OutDataType=sfix(16)  OutScaling=2^0
  In3 : Inport  Port=3  OutDataType=sfix(16)  OutScaling=2^0
  Output1 : Sum  Inputs=|+-+  OutDataType=sfix(16)  OutScaling=2^0  SaturateOnIntegerOverflow=on  InputSameDT=on
  RO : RelationalOperator  Operator=>  LogicOutDataTypeMode=boolean
  Switch : Switch  Criteria=u2 > Threshold
  Out1 : Outport  OutDataType=sfix(16)  OutScaling=2^0
  wires:
  In3/1 -> Output1/3
  Output1/1 -> Switch/1
  RO/1 -> Switch/2
  Switch/1 -> Out1/1
  In2/1 -> RO/1, Output1/1, Switch/3  "U(k)"
  In1/1 -> RO/2, Output1/2

== system MIL_Test/Test Data/Feature generation/Generate timed limited increase/Subsystem/Subsystem24 ==
  In1 : Inport  OutDataType=sfix(16)  OutScaling=2^0
  In2 : Inport  Port=2  OutDataType=sfix(16)  OutScaling=2^0
  In3 : Inport  Port=3  OutDataType=sfix(16)  OutScaling=2^0
  Output1 : Sum  Inputs=|+-+  OutDataType=sfix(16)  OutScaling=2^0  SaturateOnIntegerOverflow=on  InputSameDT=on
  RO : RelationalOperator  Operator=>  LogicOutDataTypeMode=boolean
  Switch : Switch  Criteria=u2 > Threshold
  Out1 : Outport  OutDataType=sfix(16)  OutScaling=2^0
  wires:
  In3/1 -> Output1/3
  Output1/1 -> Switch/1
  RO/1 -> Switch/2
  Switch/1 -> Out1/1
  In2/1 -> RO/1, Output1/1, Switch/3  "U(k)"
  In1/1 -> RO/2, Output1/2

== system MIL_Test/Test Data/Feature generation/Generate timed limited increase/Subsystem/Subsystem25 ==
  In1 : Inport  OutDataType=sfix(16)  OutScaling=2^0
  In2 : Inport  Port=2  OutDataType=sfix(16)  OutScaling=2^0
  In3 : Inport  Port=3  OutDataType=sfix(16)  OutScaling=2^0
  Output1 : Sum  Inputs=|+-+  OutDataType=sfix(16)  OutScaling=2^0  SaturateOnIntegerOverflow=on  InputSameDT=on
  RO : RelationalOperator  Operator=>  LogicOutDataTypeMode=boolean
  Switch : Switch  Criteria=u2 > Threshold
  Out1 : Outport  OutDataType=sfix(16)  OutScaling=2^0
  wires:
  In3/1 -> Output1/3
  Output1/1 -> Switch/1
  RO/1 -> Switch/2
  Switch/1 -> Out1/1
  In2/1 -> RO/1, Output1/1, Switch/3  "U(k)"
  In1/1 -> RO/2, Output1/2

== system MIL_Test/Test Data/Feature generation/Generate timed limited increase/Subsystem/Subsystem26 ==
  In1 : Inport  OutDataType=sfix(16)  OutScaling=2^0
  In2 : Inport  Port=2  OutDataType=sfix(16)  OutScaling=2^0
  In3 : Inport  Port=3  OutDataType=sfix(16)  OutScaling=2^0
  Output1 : Sum  Inputs=|+-+  OutDataType=sfix(16)  OutScaling=2^0  SaturateOnIntegerOverflow=on  InputSameDT=on
  RO : RelationalOperator  Operator=>  LogicOutDataTypeMode=boolean
  Switch : Switch  Criteria=u2 > Threshold
  Out1 : Outport  OutDataType=sfix(16)  OutScaling=2^0
  wires:
  In3/1 -> Output1/3
  Output1/1 -> Switch/1
  RO/1 -> Switch/2
  Switch/1 -> Out1/1
  In2/1 -> RO/1, Output1/1, Switch/3  "U(k)"
  In1/1 -> RO/2, Output1/2

== system MIL_Test/Test Data/Feature generation/Generate timed limited increase/Subsystem/Subsystem27 ==
  In1 : Inport  OutDataType=sfix(16)  OutScaling=2^0
  In2 : Inport  Port=2  OutDataType=sfix(16)  OutScaling=2^0
  In3 : Inport  Port=3  OutDataType=sfix(16)  OutScaling=2^0
  Output1 : Sum  Inputs=|+-+  OutDataType=sfix(16)  OutScaling=2^0  SaturateOnIntegerOverflow=on  InputSameDT=on
  RO : RelationalOperator  Operator=>  LogicOutDataTypeMode=boolean
  Switch : Switch  Criteria=u2 > Threshold
  Out1 : Outport  OutDataType=sfix(16)  OutScaling=2^0
  wires:
  In3/1 -> Output1/3
  Output1/1 -> Switch/1
  RO/1 -> Switch/2
  Switch/1 -> Out1/1
  In2/1 -> RO/1, Output1/1, Switch/3  "U(k)"
  In1/1 -> RO/2, Output1/2

== system MIL_Test/Test Data/Feature generation/Generate timed limited increase/Subsystem/Subsystem28 ==
  In1 : Inport  OutDataType=sfix(16)  OutScaling=2^0
  In2 : Inport  Port=2  OutDataType=sfix(16)  OutScaling=2^0
  In3 : Inport  Port=3  OutDataType=sfix(16)  OutScaling=2^0
  Output1 : Sum  Inputs=|+-+  OutDataType=sfix(16)  OutScaling=2^0  SaturateOnIntegerOverflow=on  InputSameDT=on
  RO : RelationalOperator  Operator=>  LogicOutDataTypeMode=boolean
  Switch : Switch  Criteria=u2 > Threshold
  Out1 : Outport  OutDataType=sfix(16)  OutScaling=2^0
  wires:
  In3/1 -> Output1/3
  Output1/1 -> Switch/1
  RO/1 -> Switch/2
  Switch/1 -> Out1/1
  In2/1 -> RO/1, Output1/1, Switch/3  "U(k)"
  In1/1 -> RO/2, Output1/2

== system MIL_Test/Test Data/Feature generation/Generate timed limited increase/Subsystem/Subsystem29 ==
  In1 : Inport  OutDataType=sfix(16)  OutScaling=2^0
  In2 : Inport  Port=2  OutDataType=sfix(16)  OutScaling=2^0
  In3 : Inport  Port=3  OutDataType=sfix(16)  OutScaling=2^0
  Output1 : Sum  Inputs=|+-+  OutDataType=sfix(16)  OutScaling=2^0  SaturateOnIntegerOverflow=on  InputSameDT=on
  RO : RelationalOperator  Operator=>  LogicOutDataTypeMode=boolean
  Switch : Switch  Criteria=u2 > Threshold
  Out1 : Outport  OutDataType=sfix(16)  OutScaling=2^0
  wires:
  In3/1 -> Output1/3
  Output1/1 -> Switch/1
  RO/1 -> Switch/2
  Switch/1 -> Out1/1
  In2/1 -> RO/1, Output1/1, Switch/3  "U(k)"
  In1/1 -> RO/2, Output1/2

== system MIL_Test/Test Data/Feature generation/Generate timed limited increase/Subsystem/Subsystem3 ==
  In1 : Inport  OutDataType=sfix(16)  OutScaling=2^0
  In2 : Inport  Port=2  OutDataType=sfix(16)  OutScaling=2^0
  In3 : Inport  Port=3  OutDataType=sfix(16)  OutScaling=2^0
  Output1 : Sum  Inputs=|+-+  OutDataType=sfix(16)  OutScaling=2^0  SaturateOnIntegerOverflow=on  InputSameDT=on
  RO : RelationalOperator  Operator=>  LogicOutDataTypeMode=boolean
  Switch : Switch  Criteria=u2 > Threshold
  Out1 : Outport  OutDataType=sfix(16)  OutScaling=2^0
  wires:
  In3/1 -> Output1/3
  Output1/1 -> Switch/1
  RO/1 -> Switch/2
  Switch/1 -> Out1/1
  In2/1 -> RO/1, Output1/1, Switch/3  "U(k)"
  In1/1 -> RO/2, Output1/2

== system MIL_Test/Test Data/Feature generation/Generate timed limited increase/Subsystem/Subsystem30 ==
  In1 : Inport  OutDataType=sfix(16)  OutScaling=2^0
  In2 : Inport  Port=2  OutDataType=sfix(16)  OutScaling=2^0
  In3 : Inport  Port=3  OutDataType=sfix(16)  OutScaling=2^0
  Output1 : Sum  Inputs=|+-+  OutDataType=sfix(16)  OutScaling=2^0  SaturateOnIntegerOverflow=on  InputSameDT=on
  RO : RelationalOperator  Operator=>  LogicOutDataTypeMode=boolean
  Switch : Switch  Criteria=u2 > Threshold
  Out1 : Outport  OutDataType=sfix(16)  OutScaling=2^0
  wires:
  In3/1 -> Output1/3
  Output1/1 -> Switch/1
  RO/1 -> Switch/2
  Switch/1 -> Out1/1
  In2/1 -> RO/1, Output1/1, Switch/3  "U(k)"
  In1/1 -> RO/2, Output1/2

== system MIL_Test/Test Data/Feature generation/Generate timed limited increase/Subsystem/Subsystem31 ==
  In1 : Inport  OutDataType=sfix(16)  OutScaling=2^0
  In2 : Inport  Port=2  OutDataType=sfix(16)  OutScaling=2^0
  In3 : Inport  Port=3  OutDataType=sfix(16)  OutScaling=2^0
  Output1 : Sum  Inputs=|+-+  OutDataType=sfix(16)  OutScaling=2^0  SaturateOnIntegerOverflow=on  InputSameDT=on
  RO : RelationalOperator  Operator=>  LogicOutDataTypeMode=boolean
  Switch : Switch  Criteria=u2 > Threshold
  Out1 : Outport  OutDataType=sfix(16)  OutScaling=2^0
  wires:
  In3/1 -> Output1/3
  Output1/1 -> Switch/1
  RO/1 -> Switch/2
  Switch/1 -> Out1/1
  In2/1 -> RO/1, Output1/1, Switch/3  "U(k)"
  In1/1 -> RO/2, Output1/2

== system MIL_Test/Test Data/Feature generation/Generate timed limited increase/Subsystem/Subsystem32 ==
  In1 : Inport  OutDataType=sfix(16)  OutScaling=2^0
  In2 : Inport  Port=2  OutDataType=sfix(16)  OutScaling=2^0
  In3 : Inport  Port=3  OutDataType=sfix(16)  OutScaling=2^0
  Output1 : Sum  Inputs=|+-+  OutDataType=sfix(16)  OutScaling=2^0  SaturateOnIntegerOverflow=on  InputSameDT=on
  RO : RelationalOperator  Operator=>  LogicOutDataTypeMode=boolean
  Switch : Switch  Criteria=u2 > Threshold
  Out1 : Outport  OutDataType=sfix(16)  OutScaling=2^0
  wires:
  In3/1 -> Output1/3
  Output1/1 -> Switch/1
  RO/1 -> Switch/2
  Switch/1 -> Out1/1
  In2/1 -> RO/1, Output1/1, Switch/3  "U(k)"
  In1/1 -> RO/2, Output1/2

== system MIL_Test/Test Data/Feature generation/Generate timed limited increase/Subsystem/Subsystem33 ==
  In1 : Inport  OutDataType=sfix(16)  OutScaling=2^0
  In2 : Inport  Port=2  OutDataType=sfix(16)  OutScaling=2^0
  In3 : Inport  Port=3  OutDataType=sfix(16)  OutScaling=2^0
  Output1 : Sum  Inputs=|+-+  OutDataType=sfix(16)  OutScaling=2^0  SaturateOnIntegerOverflow=on  InputSameDT=on
  RO : RelationalOperator  Operator=>  LogicOutDataTypeMode=boolean
  Switch : Switch  Criteria=u2 > Threshold
  Out1 : Outport  OutDataType=sfix(16)  OutScaling=2^0
  wires:
  In3/1 -> Output1/3
  Output1/1 -> Switch/1
  RO/1 -> Switch/2
  Switch/1 -> Out1/1
  In2/1 -> RO/1, Output1/1, Switch/3  "U(k)"
  In1/1 -> RO/2, Output1/2

== system MIL_Test/Test Data/Feature generation/Generate timed limited increase/Subsystem/Subsystem34 ==
  In1 : Inport  OutDataType=sfix(16)  OutScaling=2^0
  In2 : Inport  Port=2  OutDataType=sfix(16)  OutScaling=2^0
  In3 : Inport  Port=3  OutDataType=sfix(16)  OutScaling=2^0
  Output1 : Sum  Inputs=|+-+  OutDataType=sfix(16)  OutScaling=2^0  SaturateOnIntegerOverflow=on  InputSameDT=on
  RO : RelationalOperator  Operator=>  LogicOutDataTypeMode=boolean
  Switch : Switch  Criteria=u2 > Threshold
  Out1 : Outport  OutDataType=sfix(16)  OutScaling=2^0
  wires:
  In3/1 -> Output1/3
  Output1/1 -> Switch/1
  RO/1 -> Switch/2
  Switch/1 -> Out1/1
  In2/1 -> RO/1, Output1/1, Switch/3  "U(k)"
  In1/1 -> RO/2, Output1/2

== system MIL_Test/Test Data/Feature generation/Generate timed limited increase/Subsystem/Subsystem35 ==
  In1 : Inport  OutDataType=sfix(16)  OutScaling=2^0
  In2 : Inport  Port=2  OutDataType=sfix(16)  OutScaling=2^0
  In3 : Inport  Port=3  OutDataType=sfix(16)  OutScaling=2^0
  Output1 : Sum  Inputs=|+-+  OutDataType=sfix(16)  OutScaling=2^0  SaturateOnIntegerOverflow=on  InputSameDT=on
  RO : RelationalOperator  Operator=>  LogicOutDataTypeMode=boolean
  Switch : Switch  Criteria=u2 > Threshold
  Out1 : Outport  OutDataType=sfix(16)  OutScaling=2^0
  wires:
  In3/1 -> Output1/3
  Output1/1 -> Switch/1
  RO/1 -> Switch/2
  Switch/1 -> Out1/1
  In2/1 -> RO/1, Output1/1, Switch/3  "U(k)"
  In1/1 -> RO/2, Output1/2

== system MIL_Test/Test Data/Feature generation/Generate timed limited increase/Subsystem/Subsystem36 ==
  In1 : Inport  OutDataType=sfix(16)  OutScaling=2^0
  In2 : Inport  Port=2  OutDataType=sfix(16)  OutScaling=2^0
  In3 : Inport  Port=3  OutDataType=sfix(16)  OutScaling=2^0
  Output1 : Sum  Inputs=|+-+  OutDataType=sfix(16)  OutScaling=2^0  SaturateOnIntegerOverflow=on  InputSameDT=on
  RO : RelationalOperator  Operator=>  LogicOutDataTypeMode=boolean
  Switch : Switch  Criteria=u2 > Threshold
  Out1 : Outport  OutDataType=sfix(16)  OutScaling=2^0
  wires:
  In3/1 -> Output1/3
  Output1/1 -> Switch/1
  RO/1 -> Switch/2
  Switch/1 -> Out1/1
  In2/1 -> RO/1, Output1/1, Switch/3  "U(k)"
  In1/1 -> RO/2, Output1/2

== system MIL_Test/Test Data/Feature generation/Generate timed limited increase/Subsystem/Subsystem37 ==
  In1 : Inport  OutDataType=sfix(16)  OutScaling=2^0
  In2 : Inport  Port=2  OutDataType=sfix(16)  OutScaling=2^0
  In3 : Inport  Port=3  OutDataType=sfix(16)  OutScaling=2^0
  Output1 : Sum  Inputs=|+-+  OutDataType=sfix(16)  OutScaling=2^0  SaturateOnIntegerOverflow=on  InputSameDT=on
  RO : RelationalOperator  Operator=>  LogicOutDataTypeMode=boolean
  Switch : Switch  Criteria=u2 > Threshold
  Out1 : Outport  OutDataType=sfix(16)  OutScaling=2^0
  wires:
  In3/1 -> Output1/3
  Output1/1 -> Switch/1
  RO/1 -> Switch/2
  Switch/1 -> Out1/1
  In2/1 -> RO/1, Output1/1, Switch/3  "U(k)"
  In1/1 -> RO/2, Output1/2

== system MIL_Test/Test Data/Feature generation/Generate timed limited increase/Subsystem/Subsystem38 ==
  In1 : Inport  OutDataType=sfix(16)  OutScaling=2^0
  In2 : Inport  Port=2  OutDataType=sfix(16)  OutScaling=2^0
  In3 : Inport  Port=3  OutDataType=sfix(16)  OutScaling=2^0
  Output1 : Sum  Inputs=|+-+  OutDataType=sfix(16)  OutScaling=2^0  SaturateOnIntegerOverflow=on  InputSameDT=on
  RO : RelationalOperator  Operator=>  LogicOutDataTypeMode=boolean
  Switch : Switch  Criteria=u2 > Threshold
  Out1 : Outport  OutDataType=sfix(16)  OutScaling=2^0
  wires:
  In3/1 -> Output1/3
  Output1/1 -> Switch/1
  RO/1 -> Switch/2
  Switch/1 -> Out1/1
  In2/1 -> RO/1, Output1/1, Switch/3  "U(k)"
  In1/1 -> RO/2, Output1/2
